simulink model "LQR_BWS"  (R2023b)
settings: Solver=VariableStepAuto  StartTime=0.0  StopTime=40  RelTol=1e-3
values from neighbouring files (symbols this model uses):
  A = [0,-r/(2*J),0,0;k*r/2,0,-k/2,0;0,1/(2*m),0,0;0,0,1,0]    [LQR_bodyweight.m]
  B = [1/J,0;0,0;0,1/m;0,0]    [LQR_bodyweight.m]
  bws = .6    (= 0.6)    [LQR_bodyweight.m]
  C = eye(4)    [LQR_bodyweight.m]
  D = zeros(4,2)    [LQR_bodyweight.m]
  g = 9.81    [LQR_bodyweight.m]
  K = lqr(A2,B2,Q,R)    [LQR_bodyweight.m]
  k = 720    [LQR_bodyweight.m]
  m = 1    [LQR_bodyweight.m]
  r = .05    (= 0.05)    [LQR_bodyweight.m]
  ref = transpose(ref)    [LQR_bodyweight.m]
  Tmax = 1    [LQR_bodyweight.m]
  x0 = [0, 2*m*g*bws, 0, 0]    [LQR_bodyweight.m]
settings Model: Creator=evere  LastModifiedBy=evere

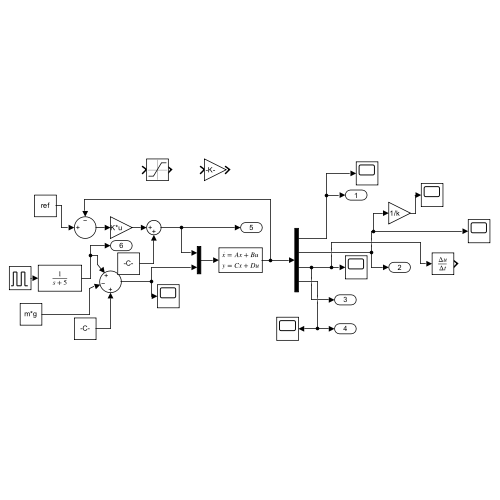
[thumbnail: Simulink's stored preview of the top-level diagram]
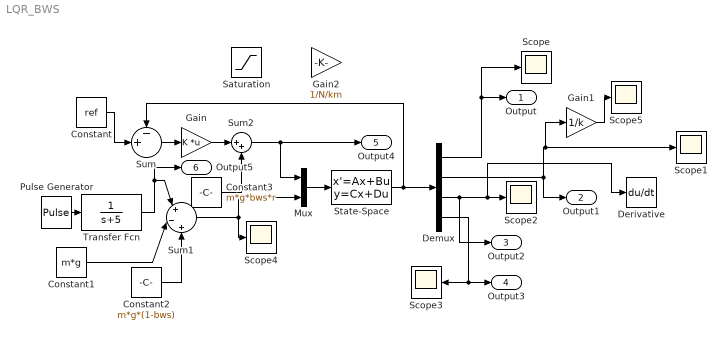
== system LQR_BWS ==
  Constant : Constant  Value=ref  VectorParams1D=off
  Constant1 : Constant  Value=m*g
  Constant2 : Constant  Value=m*g*(1-bws)
  Constant3 : Constant  Value=m*g*bws*r
  Demux : Demux
  Derivative : Derivative
  Gain : Gain  Gain=K  Multiplication=Matrix(K*u)
  Gain1 : Gain  Gain=1/k
  Gain2 : Gain  Gain=1/N/km
  Mux : Mux  Inputs=2
  Pulse Generator : DiscretePulseGenerator  PulseType=Time based  Amplitude=5  Period=10  PulseWidth=30
  Saturation : Saturate  UpperLimit=Tmax  LowerLimit=-Tmax
  Scope{,1..5} (6 alike) : Scope
  State-Space : StateSpace  A=A  B=B  C=C  D=D  InitialCondition=x0  ParameterTunability=Unconstrained
  Sum : Sum  Inputs=-+|
  Sum1 : Sum  Inputs=|+|-|+
  Sum2 : Sum  Inputs=|++
  Transfer Fcn : TransferFcn  Denominator=[1 5]
  Output : Outport
  Output1 : Outport  Port=2
  Output2 : Outport  Port=3
  Output3 : Outport  Port=4
  Output4 : Outport  Port=5
  Output5 : Outport  Port=6
  wires:
  State-Space/1 -> Sum/1, Demux/1
  Mux/1 -> State-Space/1
  Demux/2 -> Gain1/1, Scope1/1, Output1/1
  Demux/1 -> Output/1, Scope/1
  Demux/3 -> Derivative/1, Scope2/1, Output2/1
  Demux/4 -> Output3/1, Scope3/1
  Sum/1 -> Gain/1
  Constant1/1 -> Sum1/2
  Sum1/1 -> Mux/2, Scope4/1
  Gain1/1 -> Scope5/1
  Pulse Generator/1 -> Transfer Fcn/1
  Transfer Fcn/1 -> Output5/1, Sum1/1
  Constant/1 -> Sum/2
  Constant2/1 -> Sum1/3
  Constant3/1 -> Sum2/2
  Gain/1 -> Sum2/1
  Sum2/1 -> Mux/1, Output4/1
